simulink model "m_s"  (R2022b)
settings: Solver=VariableStepAuto  StartTime=0.0  StopTime=1000000  RelTol=1e-3
values from neighbouring files (symbols this model uses):
  A = J.A    [DK_iteration.m]    (also in Hinf_controller.m = Jo.A; get_linearization.m = double(subs(A, [X(1);X(2);X(3);X(4);X(5);Tau(1);Tau(2)], [x_)
  B = J.B    [DK_iteration.m]    (also in Hinf_controller.m = Jo.B; get_linearization.m = double(subs(B, [X(1);X(2);X(3);X(4);X(5);Tau(1);Tau(2)], [x_)
  C = J.C    [DK_iteration.m]    (also in Hinf_controller.m = Jo.C; get_linearization.m = double(subs(C, [X(1);X(2);X(3);X(4);X(5);Tau(1);Tau(2)], [x_)
  D = J.D    [DK_iteration.m]    (also in Hinf_controller.m = Jo.D; get_linearization.m = double(subs(D, [X(1);X(2);X(3);X(4);X(5);Tau(1);Tau(2)], [x_)
libraries: cstblocks x1
settings Model: Creator=alexi  LastModifiedBy=alexi

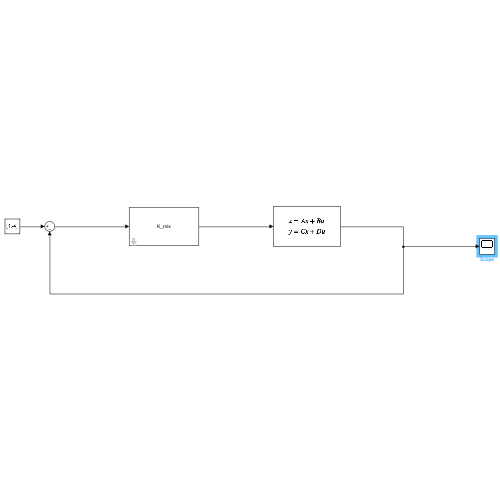
[thumbnail: Simulink's stored preview of the top-level diagram]
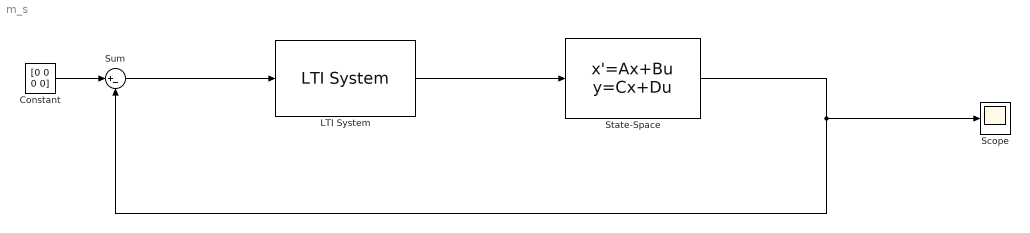
== system m_s ==
  Constant : Constant  Value=[0 0 0 0]
  LTI System : cstblocks/LTI System  sys=K_mix  IC=[]
  Scope : Scope
  State-Space : StateSpace  A=A  B=B  C=C  D=D  InitialCondition=[1 0 -0.1 0 0]  ParameterTunability=Unconstrained
  Sum : Sum  Inputs=|+-
  wires:
  Constant/1 -> Sum/1
  Sum/1 -> LTI System/1
  LTI System/1 -> State-Space/1
  State-Space/1 -> Scope/1, Sum/2
